simulink model "sampleModel1523_1_sub_sub"  (R2023a)
settings: Solver=VariableStepAuto  StartTime=0.0  StopTime=10.0  RelTol=1e-3
libraries: hdlsllib x3
settings Model: Creator=user1  LastModifiedBy=user1

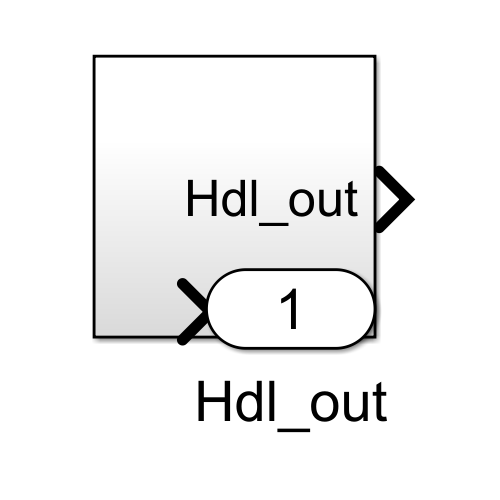
[thumbnail: Simulink's stored preview of the top-level diagram]
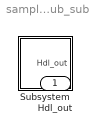
== system sampleModel1523_1_sub_sub ==
  Subsystem : Subsystem
  Hdl_out : Outport  OutDataTypeStr=uint8

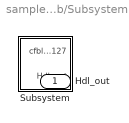
== system sampleModel1523_1_sub_sub/Subsystem ==
  Subsystem : Subsystem
  Hdl_out : Outport  OutDataTypeStr=uint8

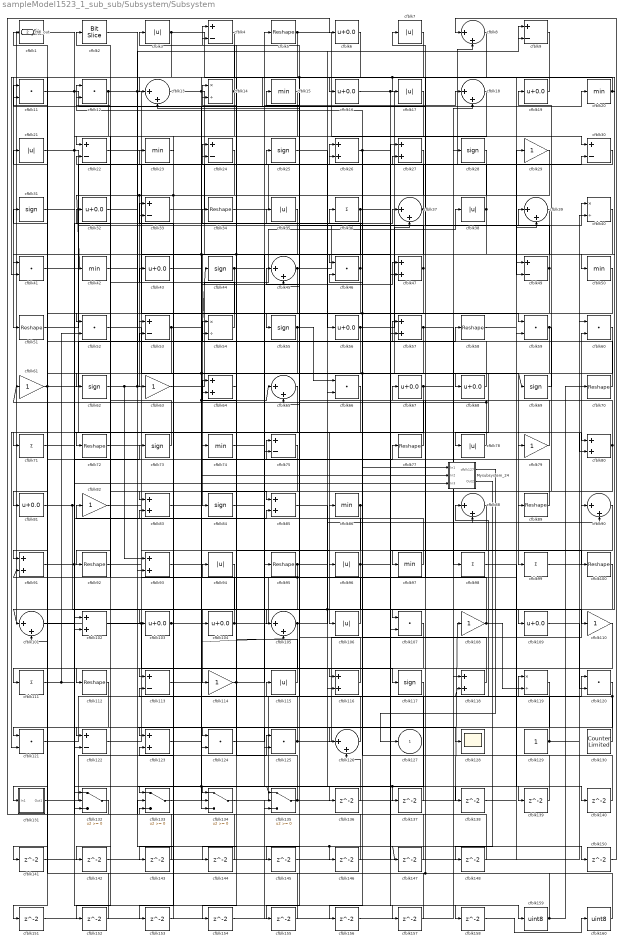
== system sampleModel1523_1_sub_sub/Subsystem/Subsystem ==
  Mysubsystem_24 : Subsystem  TreatAsAtomicUnit=on  RTWFcnName=Mysubsystem_24
      settings: RTWFcnNameOpts=User specified  RTWFileNameOpts=Use function name
  cfblk1 : hdlsllib/Logic and Bit Operations/Detect Rise Nonnegative  vinit=0  OutDataTypeStr=uint8
  cfblk{5,34,51,58,70,72,77,89,92,95,100,112} (12 alike) : Reshape
  cfblk{8,13,18,37,39,45,65,88,90,101,105,126} (12 alike) : Sum  Inputs=|++  OutDataTypeStr=uint8
  cfblk{26..27,47,57,64,80,83,85,91,93,102,116,118,123} (14 alike) : Sum  OutDataTypeStr=uint8
  cfblk{6,16,19,32,43,56,67..68,81,103..104,109} (12 alike) : Bias  Bias=0.0  SaturateOnIntegerOverflow=off
  cfblk{3,7,17,21,35,38,78,94,96,106,115} (11 alike) : Abs  OutDataTypeStr=uint8  SaturateOnIntegerOverflow=off
  cfblk{11..12,41,46,52,59..60,66,107,120..121,124..125} (13 alike) : DotProduct  OutDataTypeStr=uint8
  cfblk{29,61,63,79,82,108,110,114} (8 alike) : Gain  OutDataTypeStr=uint8
  cfblk{36,71,98..99,111} (5 alike) : Sum  Inputs=+  OutDataTypeStr=uint8
  cfblk{4,9,22,24,30,33,49,53,75,113,122} (11 alike) : Sum  Inputs=+-  OutDataTypeStr=uint8
  cfblk{25,28,31,44,55,62,69,73,84,117} (10 alike) : Signum
  cfblk{14,40,54,119} (4 alike) : Product  Inputs=*/  OutDataTypeStr=uint8  RndMeth=Zero  SaturateOnIntegerOverflow=on
  cfblk128 : Scope
  cfblk129 : Constant  OutDataTypeStr=uint8  SampleTime=-1
  cfblk130 : hdlsllib/Sources/Counter Limited  uplimit=7  tsamp=-1
  cfblk131 : Subsystem
      settings: LibrarySourceBlock=|
      | hdlsllib/Ports &
      | Subsystems/Subsystem
  cfblk{132..135} (4 alike) : Switch  OutDataTypeStr=uint8  SaturateOnIntegerOverflow=off  InputSameDT=off
  cfblk{136..148,150..158} (22 alike) : Delay  SampleTime=1
  cfblk{15,20,23,42,50,74,86,97} (8 alike) : MinMax  OutDataTypeStr=uint8
  cfblk159 : DataTypeConversion  OutDataTypeStr=uint8  SaturateOnIntegerOverflow=off  RndMeth=Floor
  cfblk160 : DataTypeConversion  OutDataTypeStr=uint8  SaturateOnIntegerOverflow=off  RndMeth=Floor
  cfblk2 : hdlsllib/Logic and Bit Operations/Bit Slice  lidx=7  ridx=0
  cfblk127 : Outport  OutDataTypeStr=uint8  VectorParamsAs1DForOutWhenUnconnected=off
  Hdl_out : Outport  Port=2  OutDataTypeStr=uint8
  wires:
  Mysubsystem_24/2(Out2) -> cfblk148/1
  Mysubsystem_24/1(cfblk127) -> cfblk127/1
  cfblk160/1 -> cfblk1/1
  cfblk158/1 -> cfblk160/1
  cfblk159/1 -> cfblk67/1, cfblk113/2, cfblk70/1
  cfblk157/1 -> cfblk53/2
  cfblk156/1 -> cfblk18/2
  cfblk155/1 -> cfblk135/2
  cfblk154/1 -> cfblk135/3
  cfblk153/1 -> cfblk123/2
  cfblk152/1 -> cfblk11/2
  cfblk119/1 -> cfblk152/1
  cfblk151/1 -> cfblk118/1
  cfblk150/1 -> cfblk8/1
  cfblk148/1 -> cfblk133/2
  cfblk147/1 -> cfblk83/2
  cfblk146/1 -> cfblk132/1
  cfblk145/1 -> cfblk57/2
  cfblk40/1 -> cfblk145/1
  cfblk144/1 -> cfblk133/3
  cfblk90/1 -> cfblk144/1
  cfblk143/1 -> cfblk102/1
  cfblk29/1 -> cfblk143/1
  cfblk142/1 -> cfblk49/1
  cfblk28/1 -> cfblk142/1
  cfblk141/1 -> cfblk60/1
  cfblk140/1 -> cfblk12/2
  cfblk98/1 -> cfblk140/1
  cfblk139/1 -> cfblk27/1
  cfblk85/1 -> cfblk139/1
  cfblk138/1 -> cfblk59/2
  cfblk84/1 -> cfblk138/1
  cfblk137/1 -> cfblk65/2
  cfblk136/1 -> cfblk126/2
  cfblk42/1 -> cfblk136/1
  cfblk130/1 -> cfblk88/1
  cfblk104/1 -> cfblk39/2, cfblk43/1
  cfblk95/1 -> cfblk123/1, cfblk91/2, cfblk9/1
  cfblk15/1 -> cfblk52/1
  cfblk66/1 -> cfblk121/2
  cfblk116/1 -> cfblk45/1
  cfblk20/1 -> cfblk13/1, cfblk50/1
  cfblk103/1 -> cfblk134/2, Hdl_out/1
  cfblk101/1 -> cfblk35/1
  cfblk110/1 -> cfblk116/1
  cfblk89/1 -> cfblk31/1
  cfblk31/1 -> cfblk33/2
  cfblk36/1 -> cfblk102/2, cfblk158/1
  cfblk120/1 -> cfblk131/1(In1), cfblk118/2
  cfblk73/1 -> cfblk2/1
  cfblk49/1 -> cfblk11/1, cfblk134/3
  cfblk133/1 -> cfblk135/1, cfblk105/2
  cfblk59/1 -> cfblk86/1, cfblk103/1, cfblk89/1
  cfblk6/1 -> cfblk104/1
  cfblk99/1 -> cfblk90/1
  cfblk44/1 -> cfblk95/1, cfblk93/2
  cfblk75/1 -> cfblk122/1
  cfblk32/1 -> cfblk26/1
  cfblk52/1 -> cfblk99/1
  cfblk121/1 -> cfblk119/1
  cfblk26/1 -> Mysubsystem_24/1(In1), cfblk100/1
  cfblk3/1 -> cfblk49/2, cfblk41/2
  cfblk107/1 -> cfblk111/1
  cfblk132/1 -> cfblk6/1
  cfblk1/1 -> cfblk159/1
  cfblk117/1 -> cfblk132/3, cfblk137/1
  cfblk111/1 -> cfblk73/1, cfblk52/2
  cfblk64/1 -> cfblk14/1
  cfblk92/1 -> cfblk96/1
  cfblk124/1 -> cfblk128/1
  cfblk33/1 -> cfblk27/2
  cfblk19/1 -> cfblk16/1
  cfblk91/1 -> cfblk85/2, cfblk107/2
  cfblk114/1 -> cfblk5/1, cfblk34/1
  cfblk80/1 -> cfblk112/1, cfblk26/2
  cfblk68/1 -> cfblk21/1
  cfblk69/1 -> cfblk19/1
  cfblk86/1 -> cfblk126/1, cfblk105/1
  cfblk23/1 -> cfblk113/1
  cfblk70/1 -> cfblk57/1
  cfblk37/1 -> cfblk23/1, cfblk154/1
  cfblk18/1 -> cfblk83/1
  cfblk54/1 -> cfblk32/1
  cfblk126/1 -> cfblk33/1
  cfblk63/1 -> cfblk38/1
  cfblk108/1 -> cfblk12/1, cfblk119/2
  cfblk56/1 -> cfblk37/2, cfblk155/1
  cfblk106/1 -> cfblk24/1
  cfblk43/1 -> cfblk85/1, cfblk69/1
  cfblk50/1 -> cfblk124/2, cfblk156/1
  cfblk30/1 -> cfblk22/2
  cfblk93/1 -> cfblk20/1
  cfblk78/1 -> cfblk61/1, cfblk13/2
  cfblk74/1 -> cfblk18/1
  cfblk34/1 -> cfblk30/2
  cfblk17/1 -> cfblk92/1
  cfblk129/1 -> cfblk40/2, cfblk14/2
  cfblk77/1 -> cfblk36/1
  cfblk5/1 -> cfblk30/1, cfblk64/2
  cfblk115/1 -> cfblk4/1
  cfblk72/1 -> cfblk74/1
  cfblk46/1 -> cfblk24/2, cfblk151/1
  cfblk55/1 -> cfblk81/1, cfblk66/1
  cfblk79/1 -> cfblk3/1
  cfblk27/1 -> cfblk42/1, cfblk53/1
  cfblk83/1 -> cfblk77/1
  cfblk51/1 -> cfblk8/2
  cfblk58/1 -> cfblk29/1
  cfblk71/1 -> cfblk110/1
  cfblk13/1 -> Mysubsystem_24/2(In2), cfblk47/2, cfblk75/2
  cfblk9/1 -> cfblk97/1
  cfblk7/1 -> cfblk55/1, cfblk41/1
  cfblk118/1 -> cfblk46/2
  cfblk21/1 -> cfblk98/1, cfblk79/1
  cfblk60/1 -> cfblk78/1
  cfblk8/1 -> cfblk17/1, cfblk45/2
  cfblk57/1 -> cfblk133/1, cfblk80/1
  cfblk123/1 -> cfblk65/1, cfblk47/1
  cfblk38/1 -> cfblk124/1, cfblk153/1, cfblk7/1
  cfblk25/1 -> cfblk56/1
  cfblk102/1 -> cfblk117/1, cfblk66/2
  cfblk113/1 -> cfblk75/1
  cfblk35/1 -> cfblk71/1
  cfblk53/1 -> cfblk44/1, cfblk122/2
  cfblk105/1 -> cfblk134/1, cfblk88/2
  cfblk14/1 -> cfblk22/1, cfblk4/2
  cfblk100/1 -> cfblk101/1, cfblk116/2
  cfblk112/1 -> cfblk121/1
  cfblk24/1 -> cfblk63/1, cfblk62/1
  cfblk135/1 -> cfblk108/1, cfblk64/1
  cfblk94/1 -> cfblk114/1
  cfblk39/1 -> cfblk84/1
  cfblk125/1 -> cfblk60/2, cfblk115/1
  cfblk96/1 -> cfblk101/2, cfblk54/1, cfblk150/1
  cfblk122/1 -> cfblk58/1
  cfblk67/1 -> cfblk106/1, cfblk90/2
  cfblk61/1 -> cfblk28/1, cfblk141/1
  cfblk12/1 -> cfblk59/1, cfblk125/2, cfblk132/2
  cfblk109/1 -> cfblk120/2
  cfblk11/1 -> cfblk109/1, cfblk157/1
  cfblk88/1 -> cfblk94/1
  cfblk47/1 -> cfblk15/1, cfblk54/2
  cfblk2/1 -> cfblk146/1, cfblk147/1
  cfblk82/1 -> cfblk37/1
  cfblk131/1(Out1) -> cfblk125/1
  cfblk22/1 -> cfblk46/1
  cfblk62/1 -> cfblk25/1, cfblk9/2, cfblk93/1
  cfblk81/1 -> Mysubsystem_24/3(In3), cfblk107/1
  cfblk4/1 -> cfblk51/1
  cfblk45/1 -> cfblk40/1, cfblk91/1
  cfblk134/1 -> cfblk120/1
  cfblk16/1 -> cfblk68/1, cfblk80/2
  cfblk65/1 -> cfblk72/1
  cfblk97/1 -> cfblk82/1
  cfblk41/1 -> cfblk39/1

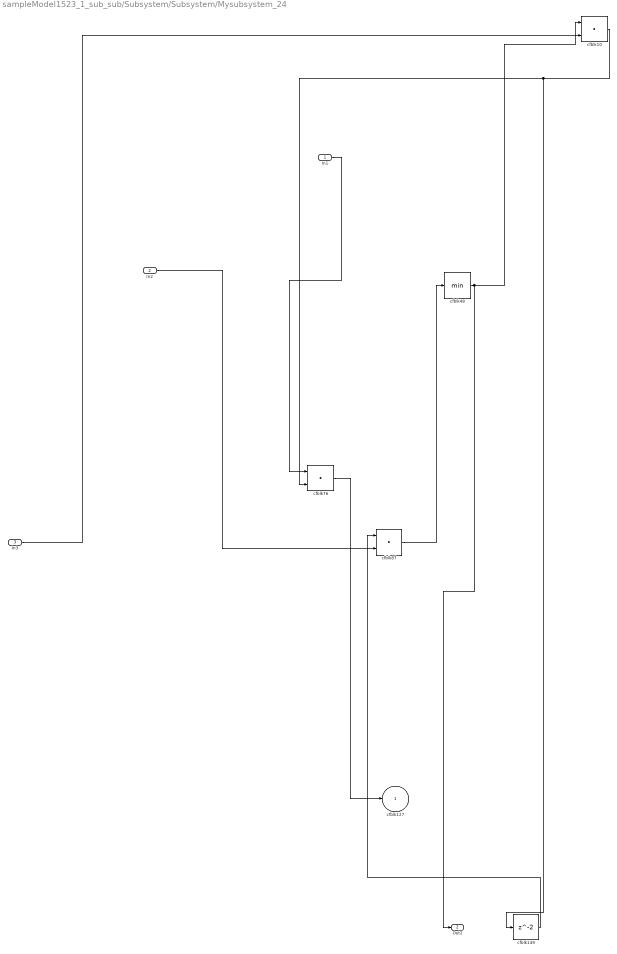
== system sampleModel1523_1_sub_sub/Subsystem/Subsystem/Mysubsystem_24 ==
  In1 : Inport
  In2 : Inport  Port=2
  In3 : Inport  Port=3
  cfblk10 : DotProduct  OutDataTypeStr=Inherit: Inherit via internal rule
  cfblk149 : Delay  SampleTime=1
  cfblk48 : MinMax
  cfblk76 : DotProduct  OutDataTypeStr=Inherit: Inherit via internal rule
  cfblk87 : DotProduct  OutDataTypeStr=Inherit: Inherit via internal rule
  cfblk127 : Outport  VectorParamsAs1DForOutWhenUnconnected=off
  Out2 : Outport  Port=2
  wires:
  cfblk149/1 -> cfblk87/1
  cfblk10/1 -> cfblk76/2, cfblk149/1
  In1/1 -> cfblk76/1
  cfblk48/1 -> Out2/1, cfblk10/1
  In2/1 -> cfblk87/2
  cfblk87/1 -> cfblk48/1
  cfblk76/1 -> cfblk127/1
  In3/1 -> cfblk10/2

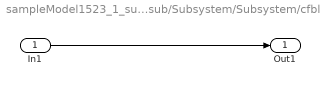
== system sampleModel1523_1_sub_sub/Subsystem/Subsystem/cfblk131 ==
  In1 : Inport
  Out1 : Outport
  wires:
  In1/1 -> Out1/1
